simulink model "rpi_arduino_rw"  (R2018b)
settings: Solver=FixedStepAuto  StartTime=0.0  StopTime=inf  RelTol=1e-3  EnableMultiTasking=on
libraries: raspberrypilib x5, sensehatlib x1
settings Model: SimulationMode=external  Creator=mnimi  LastModifiedBy=mnimi
settings SolverCC: PositivePriorityOrder=on
settings OptimizationCC: EnhancedBackFolding=on  PassReuseOutputArgsAs=Individual arguments  MaxStackSize=64  OptimizeBlockOrder=speed  DifferentSizesBufferReuse=on  OptimizationCustomize=off
settings DebuggingCC: ParameterTunabilityLossMsg=error
settings HardwareCC: ProdBitPerPointer=32  ProdBitPerSizeT=32  ProdBitPerPtrDiffT=32  ProdLargestAtomicInteger=Long  ProdLargestAtomicFloat=Double  ProdWordSize=32  ProdHWDeviceType=ARM Compatible->ARM Cortex
settings ModelReferenceCC: UpdateModelReferenceTargets=Force
settings SFSimCC: MATLABDynamicMemAlloc=off
settings RTWCC: SystemTargetFile=ert.tlc  HardwareBoard=Raspberry Pi  TLCOptions="-aInlineSetEventsForThisBaseRateFcn=TLC_FALSE -aSuppressMultiTaskScheduler=TLC_FALSE  -aRateBasedStepFcn=0"  TemplateMakefile=ert_default_tmf  GenerateReport=on  Toolchain=GNU GCC Raspberry Pi  BuildConfiguration=Faster Runs  IncludeHyperlinkInReport=on  LaunchReport=on  GenerateTraceInfo=on  GenerateTraceReport=on  GenerateTraceReportSl=on  GenerateTraceReportSf=on  GenerateTraceReportEml=on
settings CodeAppCC: ForceParamTrailComments=on  IgnoreCustomStorageClasses=off  OperatorAnnotations=on  SimulinkDataObjDesc=on  SFDataObjDesc=on  InsertBlockDesc=on
settings ERTTargetCC: SupportVariableSizeSignals=on

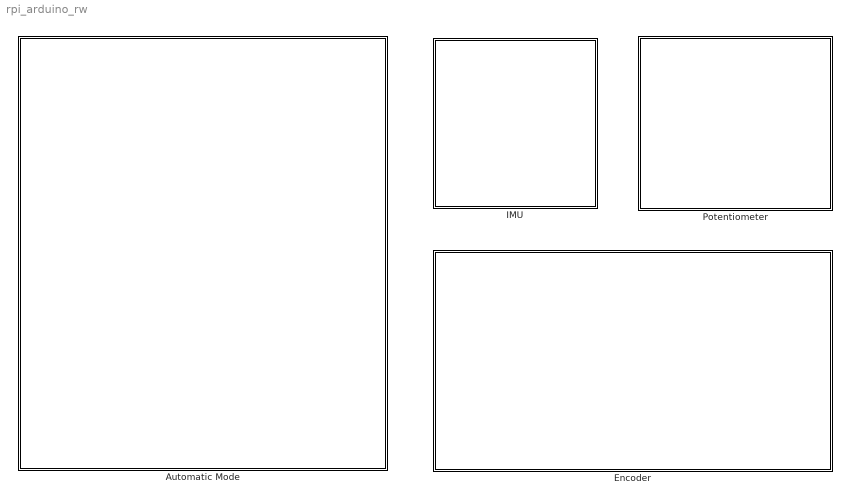
== system rpi_arduino_rw ==
  Automatic Mode : Subsystem
  Encoder : Subsystem
  IMU : Subsystem
  Potentiometer : Subsystem

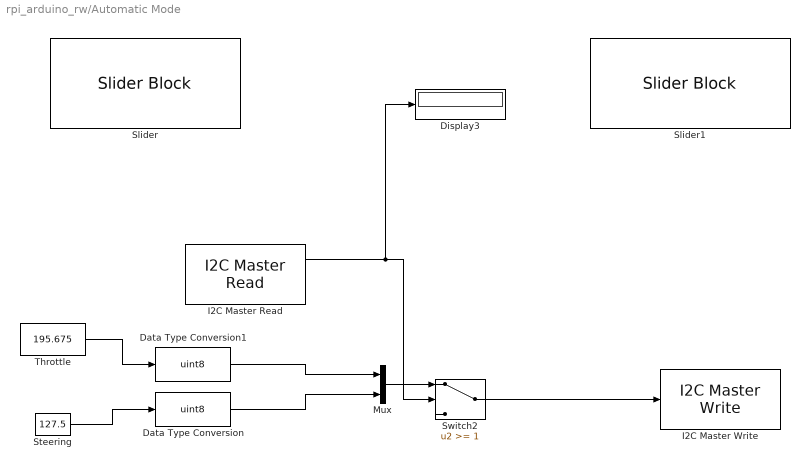
== system rpi_arduino_rw/Automatic Mode ==
  Data Type Conversion : DataTypeConversion  OutDataTypeStr=uint8
  Data Type Conversion1 : DataTypeConversion  OutDataTypeStr=uint8
  Display3 : Display
  I2C Master Read : raspberrypilib/I2C Master Read  BoardProperty=Pi 3 Model B+  Mode=Master  SlaveAddress=1  SlaveByteOrder=LittleEndian  Direction=Receiver  RegisterAddressMode=off  RegisterAddress=0  SlaveDataType=uint8  DataLength=1  NoAck=off  RepeatedStart=off  OutputStatus=on  SampleTime=0.1
      settings: SourceProductName=Simulink Support Package for Raspberry Pi Hardware  SourceProductBaseCode=RASPPI
  I2C Master Write : raspberrypilib/I2C Master Write  BoardProperty=Pi 3 Model B+  Mode=Master  SlaveAddress=1  SlaveByteOrder=LittleEndian  Direction=Transmitter  RegisterAddressMode=off  RegisterAddress=0  SlaveDataType=uint8  DataLength=1  NoAck=off  RepeatedStart=off  OutputStatus=off
      settings: SourceProductName=Simulink Support Package for Raspberry Pi Hardware  SourceProductBaseCode=RASPPI
  Mux : Mux  Inputs=2
  Slider : SliderBlock  WebBlockId=45  ScaleMin=189  ScaleMax=197
  Slider1 : SliderBlock  WebBlockId=46  ScaleMin=127.5  ScaleMax=255
  Steering : Constant  Value=127.5
  Switch2 : Switch  Threshold=1
  Throttle : Constant  Value=195.675
  wires:
  Data Type Conversion/1 -> Mux/2
  I2C Master Read/1 -> Display3/1, Switch2/2
  Data Type Conversion1/1 -> Mux/1
  Steering/1 -> Data Type Conversion/1
  Throttle/1 -> Data Type Conversion1/1
  Mux/1 -> Switch2/1
  Switch2/1 -> I2C Master Write/1

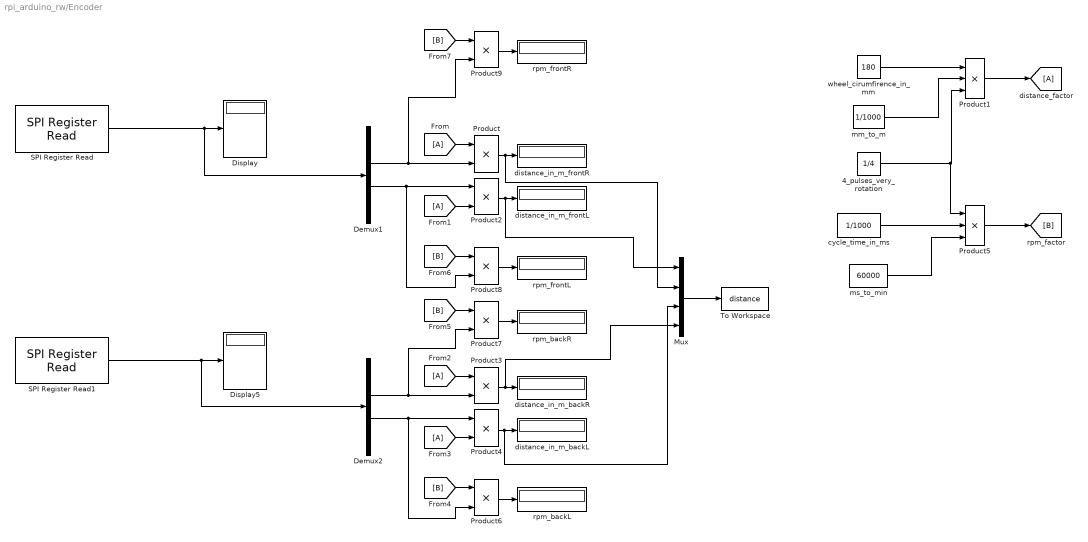
== system rpi_arduino_rw/Encoder ==
  4_pulses_very_rotation : Constant  Value=1/4
  Demux1 : Demux
  Demux2 : Demux
  Display : Display
  Display5 : Display
  Mux : Mux
  Product{,2..4,6..9} (8 alike) : Product
  Product1 : Product  Inputs=3
  Product5 : Product  Inputs=3
  SPI Register Read : raspberrypilib/SPI Register Read  BoardProperty=Pi 3 Model B+  SPIModule=uint32(0)  Mode=Master  BusSpeed=1000000  Pin=SPI0_CE0  FirstBitToTransfer=Most significant bit (MSB)  ClockMode=0  BlockFunction=Read  RegisterAddress=0  OutputDataType=uint8  OutputDataLength=4  SampleTime=1
      settings: SourceProductName=Simulink Support Package for Raspberry Pi Hardware  SourceProductBaseCode=RASPPI
  SPI Register Read1 : raspberrypilib/SPI Register Read  BoardProperty=Pi 3 Model B+  SPIModule=uint32(0)  Mode=Master  BusSpeed=1000000  Pin=SPI0_CE1  FirstBitToTransfer=Most significant bit (MSB)  ClockMode=0  BlockFunction=Read  RegisterAddress=0  OutputDataType=uint8  OutputDataLength=4  SampleTime=1
      settings: SourceProductName=Simulink Support Package for Raspberry Pi Hardware  SourceProductBaseCode=RASPPI
  To Workspace : ToWorkspace  VariableName=distance  SampleTime=-1
      settings: Save2DSignal=2-D array (concatenate along first dimension)
  cycle_time_in_ms : Constant  Value=1/1000
  distance_in_m_backL : Display
  distance_in_m_backR : Display
  distance_in_m_frontL : Display
  distance_in_m_frontR : Display
  mm_to_m : Constant  Value=1/1000
  ms_to_min : Constant  Value=60000
  rpm_backL : Display
  rpm_backR : Display
  rpm_frontL : Display
  rpm_frontR : Display
  wheel_cirumfirence_in_mm : Constant  Value=180
  wires:
  cycle_time_in_ms/1 -> Product5/2
  Demux2/2 -> Product7/2, Product3/2
  [B] -> Product9/1
  [A] -> Product3/1
  [A] -> Product4/2
  Product/1 -> Mux/2, distance_in_m_frontR/1
  Demux1/3 -> Product8/2, Product2/1
  [A] -> Product/1
  4_pulses_very_rotation/1 -> Product5/1, Product1/3
  [B] -> Product6/1
  Demux1/2 -> Product9/2, Product/2
  SPI Register Read1/1 -> Display5/1, Demux2/1
  wheel_cirumfirence_in_mm/1 -> Product1/1
  mm_to_m/1 -> Product1/2
  Product8/1 -> rpm_frontL/1
  Product4/1 -> Mux/3, distance_in_m_backL/1
  SPI Register Read/1 -> Display/1, Demux1/1
  Product7/1 -> rpm_backR/1
  [B] -> Product8/1
  Product2/1 -> Mux/1, distance_in_m_frontL/1
  Product6/1 -> rpm_backL/1
  [B] -> Product7/1
  Demux2/3 -> Product6/2, Product4/1
  [A] -> Product2/2
  Product9/1 -> rpm_frontR/1
  Product3/1 -> Mux/4, distance_in_m_backR/1
  Product5/1 -> [B]
  ms_to_min/1 -> Product5/3
  Product1/1 -> [A]
  Mux/1 -> To Workspace/1

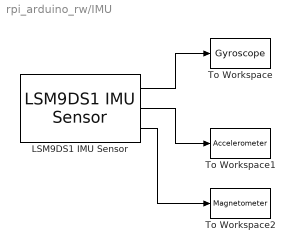
== system rpi_arduino_rw/IMU ==
  LSM9DS1 IMU Sensor : sensehatlib/LSM9DS1 IMU Sensor  blockPlatform=Raspberry Pi  BoardProperty_sh=Pi 3 Model B  ActiveSensors_=Accelerometer, Gyroscope and Magnetometer  AccelerometerOutputDataRate=119 Hz  AccelerometerFullScaleRange=+/- 2g  AccelerometerBandwidth=50 Hz  GyroscopeOutputDataRate=119 Hz  GyroscopeFullScaleRange=245 dps  GyroscopeBandwidthMode=0  GyroscopeHighPassFilterEnabled=off  GyroscopeHighPassFilterMode=0  MagnetometerFullScaleRange=+/- 4 gauss  MagnetometerOutputDataRate=40 Hz  SampleTime=0.1
      settings: SourceProductName=Simulink Support Package for Raspberry Pi Hardware  SourceProductBaseCode=RASPPI
  To Workspace : ToWorkspace  VariableName=Gyroscope  SampleTime=-1
      settings: Save2DSignal=2-D array (concatenate along first dimension)
  To Workspace1 : ToWorkspace  VariableName=Accelerometer  SampleTime=-1
      settings: Save2DSignal=2-D array (concatenate along first dimension)
  To Workspace2 : ToWorkspace  VariableName=Magnetometer  SampleTime=-1
      settings: Save2DSignal=2-D array (concatenate along first dimension)
  wires:
  LSM9DS1 IMU Sensor/2 -> To Workspace1/1
  LSM9DS1 IMU Sensor/1 -> To Workspace/1
  LSM9DS1 IMU Sensor/3 -> To Workspace2/1

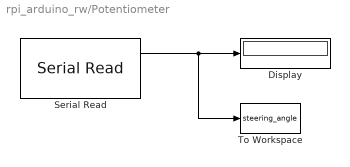
== system rpi_arduino_rw/Potentiometer ==
  Display : Display
  Serial Read : raspberrypilib/Serial Read  board=Pi 3 Model B  SCIModule_=/dev/ttyUSB0  Baudrate_=9600  Parity=None  StopBits_=1  HardwareFlowControl=None  ByteOrder=LittleEndian  DataLength=1  DataType=int8  OutputStatus=on  SampleTime=0.01  blockPlatform=RaspberryPi
      settings: SourceProductName=Simulink Support Package for Raspberry Pi Hardware  SourceProductBaseCode=RASPPI
  To Workspace : ToWorkspace  VariableName=steering_angle  SampleTime=-1
      settings: Save2DSignal=2-D array (concatenate along first dimension)
  wires:
  Serial Read/1 -> To Workspace/1, Display/1
